simulink model "LAB_04_17_OCT_SIM_KIN_QUAT"  (R2022b)
settings: Solver=ode4  StartTime=0.0  StopTime=100  FixedStep=0.1  RelTol=1e-3
values from neighbouring files (symbols this model uses):
  I = [Ix 0 0 ... (first row only)    [LAB_03_3_OCT_MAT_EUL_2_VERIFICATION.m]    (also in LAB_03_3_OCT_MAT_EUL_DOUBLESPIN.m = diag([Ix, Iy, Iz]); LAB_03_3_OCT_MAT_EUL_SPINAXIS.m = diag([Ix, Iy, Iz]); LAB_03_3_OCT_MAT_EUL_VECT.m; LAB_04_17_OCT_MAT_KIN.m)
  om_0 = [om_x0, om_y0, om_z0]    [LAB_03_3_OCT_MAT_EUL.m]    (also in LAB_03_3_OCT_MAT_EUL_2_VERIFICATION.m = [om_x0; om_y0; om_z0]; LAB_03_3_OCT_MAT_EUL_DOUBLESPIN.m = [om_x0; om_y0; om_z0]; LAB_03_3_OCT_MAT_EUL_SPINAXIS.m = [om_x0; om_y0; om_z0]; LAB_03_3_OCT_MAT_EUL_VECT.m = [om_x0; om_y0; om_z0])
  q0 = [0, 0, 0, 1]'    [LAB_04_17_OCT_MAT_KIN.m]    (also in core_attitude_test.m = [0;0;0;1])
libraries: sharedutil x1, matrix_library x1
settings Model: Creator=maria  LastModifiedBy=maria

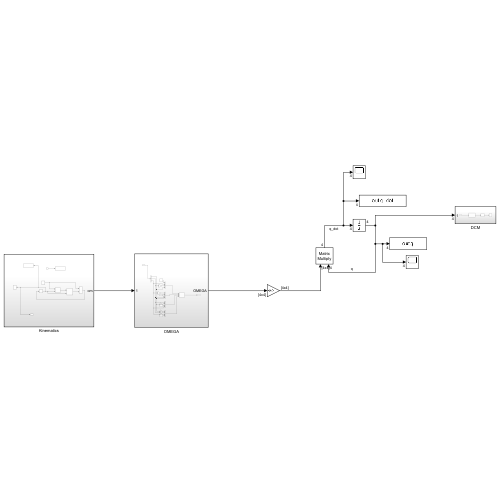
[thumbnail: Simulink's stored preview of the top-level diagram]
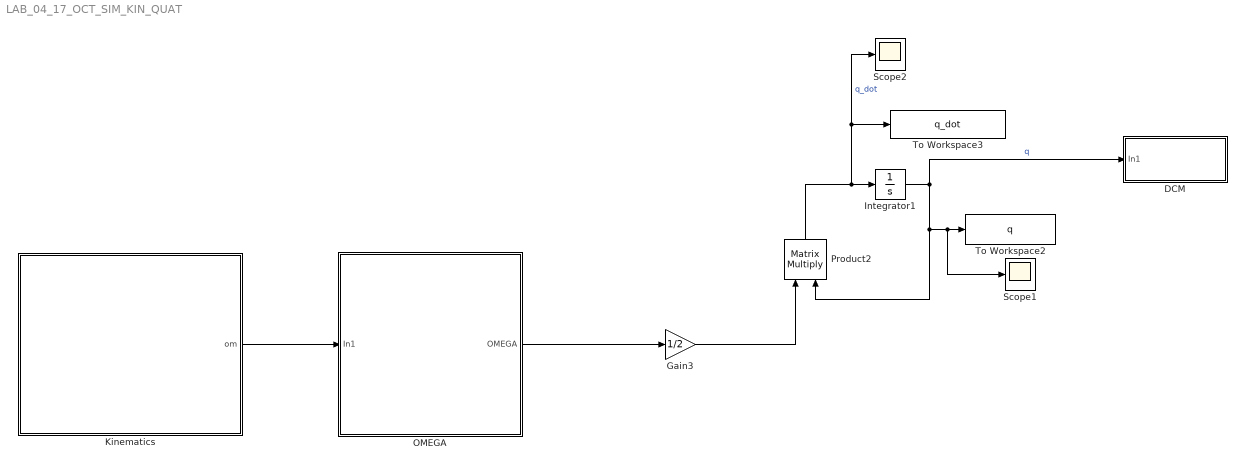
== system LAB_04_17_OCT_SIM_KIN_QUAT ==
  DCM : Subsystem
  Gain3 : Gain  Gain=1/2
  Integrator1 : Integrator  InitialCondition=q0
  Kinematics : Subsystem
  OMEGA : Subsystem
  Product2 : Product  Multiplication=Matrix(*)
  Scope1 : Scope
  Scope2 : Scope
  To Workspace2 : ToWorkspace  VariableName=q  SaveFormat=Timeseries  SampleTime=-1
  To Workspace3 : ToWorkspace  VariableName=q_dot  SaveFormat=Timeseries  SampleTime=-1
  wires:
  Gain3/1 -> Product2/1
  Integrator1/1 -> Product2/2, Scope1/1, To Workspace2/1, DCM/1(In1)  "q"
  Product2/1 -> Scope2/1, To Workspace3/1, Integrator1/1  "q_dot"
  Kinematics/1(om) -> OMEGA/1(In1)
  OMEGA/1(OMEGA) -> Gain3/1

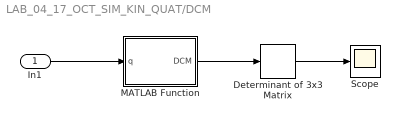
== system LAB_04_17_OCT_SIM_KIN_QUAT/DCM ==
  In1 : Inport
  Determinant of 3x3 Matrix : sharedutil/Determinant of 3x3 Matrix  aMode=aMode
      settings: LibrarySourceBlock=|
      | aerolibutil/Determinant of
      | 3x3 Matrix
  MATLAB Function : MATLAB Function  TreatAsAtomicUnit=on
  Scope : Scope
  wires:
  In1/1 -> MATLAB Function/1(q)
  MATLAB Function/1(DCM) -> Determinant of 3x3 Matrix/1
  Determinant of 3x3 Matrix/1 -> Scope/1

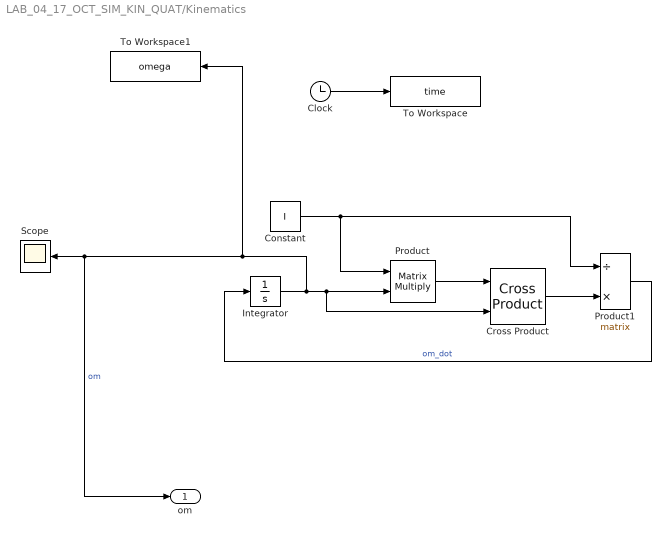
== system LAB_04_17_OCT_SIM_KIN_QUAT/Kinematics ==
  Clock : Clock
  Constant : Constant  Value=I
  Cross Product : matrix_library/Cross Product
  Integrator : Integrator  InitialCondition=om_0
  Product : Product  Multiplication=Matrix(*)
  Product1 : Product  Inputs=/*  Multiplication=Matrix(*)
  Scope : Scope
  To Workspace : ToWorkspace  VariableName=time  SaveFormat=Timeseries  SampleTime=-1
  To Workspace1 : ToWorkspace  VariableName=omega  SampleTime=-1
  om : Outport
  wires:
  Integrator/1 -> To Workspace1/1, om/1, Scope/1, Product/2, Cross Product/2  "om"
  Cross Product/1 -> Product1/2
  Product/1 -> Cross Product/1
  Constant/1 -> Product/1, Product1/1
  Product1/1 -> Integrator/1  "om_dot"
  Clock/1 -> To Workspace/1

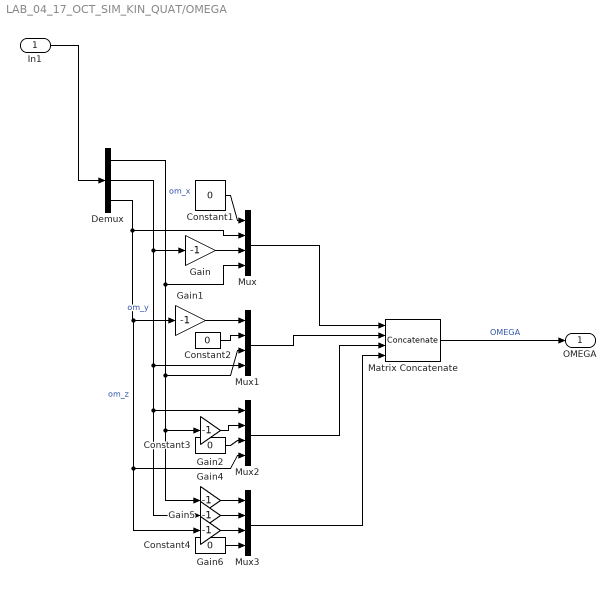
== system LAB_04_17_OCT_SIM_KIN_QUAT/OMEGA ==
  In1 : Inport
  Constant{1..4} (4 alike) : Constant  Value=0
  Demux : Demux  Outputs=3
  Gain{,1..2,4..6} (6 alike) : Gain  Gain=-1
  Matrix Concatenate : Concatenate  NumInputs=4  Mode=Multidimensional array  ConcatenateDimension=2
  Mux{,1..3} (4 alike) : Mux
  OMEGA : Outport
  wires:
  Mux/1 -> Matrix Concatenate/1
  Constant2/1 -> Mux1/2
  Matrix Concatenate/1 -> OMEGA/1  "OMEGA"
  Constant4/1 -> Mux3/4
  Mux1/1 -> Matrix Concatenate/2
  Mux2/1 -> Matrix Concatenate/3
  Constant1/1 -> Mux/1
  Constant3/1 -> Mux2/3
  Demux/3 -> Mux/2, Gain6/1, Mux2/4, Gain1/1  "om_z"
  Gain2/1 -> Mux2/2
  Demux/2 -> Gain5/1, Mux2/1, Mux1/4, Gain/1  "om_y"
  Gain6/1 -> Mux3/3
  Mux3/1 -> Matrix Concatenate/4
  Demux/1 -> Mux/4, Mux1/3, Gain4/1, Gain2/1  "om_x"
  Gain4/1 -> Mux3/1
  Gain/1 -> Mux/3
  Gain1/1 -> Mux1/1
  Gain5/1 -> Mux3/2
  In1/1 -> Demux/1

== matlab function LAB_04_17_OCT_SIM_KIN_QUAT/DCM/MATLAB Function ==
  data: q input; DCM output
function DCM = fcn(q)

q1 = q(1);
q2 = q(2);
q3 = q(3);
q4 = q(4);

DCM = [q1^2-q2^2-q3^2+q4^2, 2*(q1*q2+q3*q4), 2*(q1*q3-q2*q4);
        2*(q1*q2-q3*q4), -q1^2+q2^2-q3^2+q4^2, 2*(q2*q3+q1*q4);
        2*(q1*q3+q2*q4), 2*(q2*q3-q1*q4), -q1^2-q2^2+q3^2+q4^2];

end
